simulink library "topr5_adapter"  (Simulink 8.2)
settings: Solver=ode1  StartTime=0.0  StopTime=Inf  FixedStep=0.001  RelTol=1e-3
PostLoadFcn:
  | , if any(exist('dsrtsu_mdlpostloadfcn', 'file') == [2, 3, 6]), try dsrtsu_mdlpostloadfcn('Execute', bdroot); catch fprintf('Error in PostLoadFcn (dsrtsu_mdlpostloadfcn) for model "%s":\n %s\n', bdroot, lasterr); end, end,
libraries: ParsingLibrary x32, simulink x4, srx_platform x3, topr5_adapter x2
settings Model: DSRTSU_INTERNAL_RTI_VER=450  DSRTSU_INTERNAL_RTI_TYPE=rti1401  DSRTSU_INTERNAL_RTIFPGA=40  Creator=leidos  LastModifiedBy=rushk1

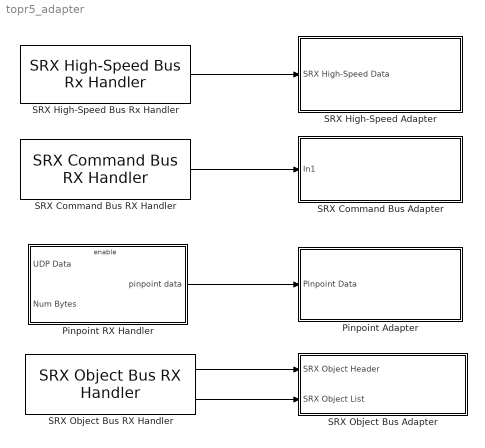
== system topr5_adapter ==
  Pinpoint Adapter : Subsystem
  Pinpoint RX Handler : Subsystem
  SRX Command Bus Adapter : Subsystem
  SRX Command Bus RX Handler : srx_platform/SRX Command Bus RX Handler  SystemSampleTime=-1
  SRX High-Speed Adapter : Subsystem
  SRX High-Speed Bus Rx Handler : srx_platform/SRX High-Speed Bus Rx Handler  SystemSampleTime=-1
  SRX Object Bus Adapter : Subsystem
  SRX Object Bus RX Handler : srx_platform/SRX Object Bus RX Handler
  wires:
  SRX Command Bus RX Handler/1 -> SRX Command Bus Adapter/1(In1)
  SRX High-Speed Bus Rx Handler/1 -> SRX High-Speed Adapter/1(SRX High-Speed Data)
  Pinpoint RX Handler/1(pinpoint data) -> Pinpoint Adapter/1(Pinpoint Data)
  SRX Object Bus RX Handler/1 -> SRX Object Bus Adapter/1(SRX Object Header)
  SRX Object Bus RX Handler/2 -> SRX Object Bus Adapter/2(SRX Object List)

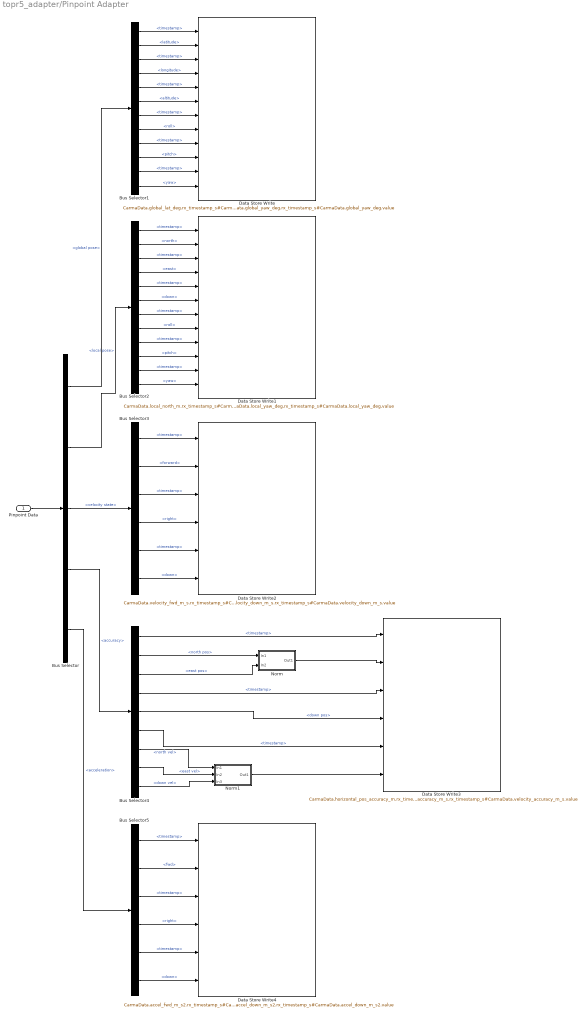
== system topr5_adapter/Pinpoint Adapter ==
  Pinpoint Data : Inport
  Bus Selector : BusSelector  OutputSignals=global pose,local pose,velocity state,accuracy,acceleration
  Bus Selector1 : BusSelector  OutputSignals=timestamp,latitude,timestamp,longitude,timestamp,altitude,timestamp,roll,timestamp,pitch,timestamp,yaw
  Bus Selector2 : BusSelector  OutputSignals=timestamp,north,timestamp,east,timestamp,down,timestamp,roll,timestamp,pitch,timestamp,yaw
  Bus Selector3 : BusSelector  OutputSignals=timestamp,forward,timestamp,right,timestamp,down
  Bus Selector4 : BusSelector  OutputSignals=timestamp,north pos,east pos,timestamp,down pos,timestamp,north vel,east vel,down vel
  Bus Selector5 : BusSelector  OutputSignals=timestamp,fwd,timestamp,right,timestamp,down
  Data Store Write : DataStoreWrite  DataStoreName=CarmaData  DataStoreElements=CarmaData.global_lat_deg.rx_timestamp_s#CarmaData.global_lat_deg.value#CarmaData.global_long_deg.rx_timestamp_s#CarmaData.global_long_deg.value#CarmaData.global_alt_m.rx_timestamp_s#CarmaData.global_alt_m.value#CarmaData.global_roll_deg.rx_timestamp_s#CarmaData.global_roll_deg.value#CarmaData.global_pitch_deg.rx_timestamp_s#CarmaData.global_pitch_deg.value#CarmaData.global_yaw_deg.rx_timestamp_s#CarmaData.global_yaw_deg.value
  Data Store Write1 : DataStoreWrite  DataStoreName=CarmaData  DataStoreElements=CarmaData.local_north_m.rx_timestamp_s#CarmaData.local_north_m.value#CarmaData.local_east_m.rx_timestamp_s#CarmaData.local_east_m.value#CarmaData.local_down_m.rx_timestamp_s#CarmaData.local_down_m.value#CarmaData.local_roll_deg.rx_timestamp_s#CarmaData.local_roll_deg.value#CarmaData.local_pitch_deg.rx_timestamp_s#CarmaData.local_pitch_deg.value#CarmaData.local_yaw_deg.rx_timestamp_s#CarmaData.local_yaw_deg.value
  Data Store Write2 : DataStoreWrite  DataStoreName=CarmaData  DataStoreElements=CarmaData.velocity_fwd_m_s.rx_timestamp_s#CarmaData.velocity_fwd_m_s.value#CarmaData.velocity_right_m_s.rx_timestamp_s#CarmaData.velocity_right_m_s.value#CarmaData.velocity_down_m_s.rx_timestamp_s#CarmaData.velocity_down_m_s.value
  Data Store Write3 : DataStoreWrite  DataStoreName=CarmaData  DataStoreElements=CarmaData.horizontal_pos_accuracy_m.rx_timestamp_s#CarmaData.horizontal_pos_accuracy_m.value#CarmaData.vertical_pos_accuracy_m.rx_timestamp_s#CarmaData.vertical_pos_accuracy_m.value#CarmaData.velocity_accuracy_m_s.rx_timestamp_s#CarmaData.velocity_accuracy_m_s.value
  Data Store Write4 : DataStoreWrite  DataStoreName=CarmaData  DataStoreElements=CarmaData.accel_fwd_m_s2.rx_timestamp_s#CarmaData.accel_fwd_m_s2.value#CarmaData.accel_right_m_s2.rx_timestamp_s#CarmaData.accel_right_m_s2.value#CarmaData.accel_down_m_s2.rx_timestamp_s#CarmaData.accel_down_m_s2.value
  Norm : Subsystem
  Norm1 : Subsystem
  wires:
  Bus Selector1/5 -> Data Store Write/5  "<timestamp>"
  Bus Selector1/3 -> Data Store Write/3  "<timestamp>"
  Bus Selector1/2 -> Data Store Write/2  "<latitude>"
  Bus Selector1/9 -> Data Store Write/9  "<timestamp>"
  Bus Selector1/6 -> Data Store Write/6  "<altitude>"
  Bus Selector1/7 -> Data Store Write/7  "<timestamp>"
  Bus Selector1/8 -> Data Store Write/8  "<roll>"
  Bus Selector1/11 -> Data Store Write/11  "<timestamp>"
  Bus Selector1/1 -> Data Store Write/1  "<timestamp>"
  Bus Selector1/4 -> Data Store Write/4  "<longitude>"
  Bus Selector1/10 -> Data Store Write/10  "<pitch>"
  Bus Selector1/12 -> Data Store Write/12  "<yaw>"
  Bus Selector5/3 -> Data Store Write4/3  "<timestamp>"
  Bus Selector5/2 -> Data Store Write4/2  "<fwd>"
  Bus Selector5/4 -> Data Store Write4/4  "<right>"
  Bus Selector5/6 -> Data Store Write4/6  "<down>"
  Bus Selector5/1 -> Data Store Write4/1  "<timestamp>"
  Bus Selector5/5 -> Data Store Write4/5  "<timestamp>"
  Bus Selector/5 -> Bus Selector5/1  "<acceleration>"
  Bus Selector4/6 -> Data Store Write3/5  "<timestamp>"
  Bus Selector4/5 -> Data Store Write3/4  "<down pos>"
  Bus Selector4/4 -> Data Store Write3/3  "<timestamp>"
  Bus Selector4/1 -> Data Store Write3/1  "<timestamp>"
  Bus Selector/4 -> Bus Selector4/1  "<accuracy>"
  Bus Selector3/6 -> Data Store Write2/6  "<down>"
  Bus Selector3/5 -> Data Store Write2/5  "<timestamp>"
  Bus Selector3/1 -> Data Store Write2/1  "<timestamp>"
  Bus Selector3/2 -> Data Store Write2/2  "<forward>"
  Bus Selector3/4 -> Data Store Write2/4  "<right>"
  Bus Selector3/3 -> Data Store Write2/3  "<timestamp>"
  Bus Selector/3 -> Bus Selector3/1  "<velocity state>"
  Bus Selector2/3 -> Data Store Write1/3  "<timestamp>"
  Bus Selector2/11 -> Data Store Write1/11  "<timestamp>"
  Bus Selector2/9 -> Data Store Write1/9  "<timestamp>"
  Bus Selector2/7 -> Data Store Write1/7  "<timestamp>"
  Bus Selector2/12 -> Data Store Write1/12  "<yaw>"
  Bus Selector2/5 -> Data Store Write1/5  "<timestamp>"
  Bus Selector2/6 -> Data Store Write1/6  "<down>"
  Bus Selector2/10 -> Data Store Write1/10  "<pitch>"
  Bus Selector2/8 -> Data Store Write1/8  "<roll>"
  Bus Selector2/4 -> Data Store Write1/4  "<east>"
  Bus Selector2/1 -> Data Store Write1/1  "<timestamp>"
  Bus Selector2/2 -> Data Store Write1/2  "<north>"
  Bus Selector/2 -> Bus Selector2/1  "<local pose>"
  Bus Selector/1 -> Bus Selector1/1  "<global pose>"
  Pinpoint Data/1 -> Bus Selector/1
  Norm1/1(Out1) -> Data Store Write3/6
  Bus Selector4/2 -> Norm/1(In1)  "<north pos>"
  Bus Selector4/3 -> Norm/2(In2)  "<east pos>"
  Norm/1(Out1) -> Data Store Write3/2
  Bus Selector4/7 -> Norm1/1(In1)  "<north vel>"
  Bus Selector4/8 -> Norm1/2(In2)  "<east vel>"
  Bus Selector4/9 -> Norm1/3(In3)  "<down vel>"

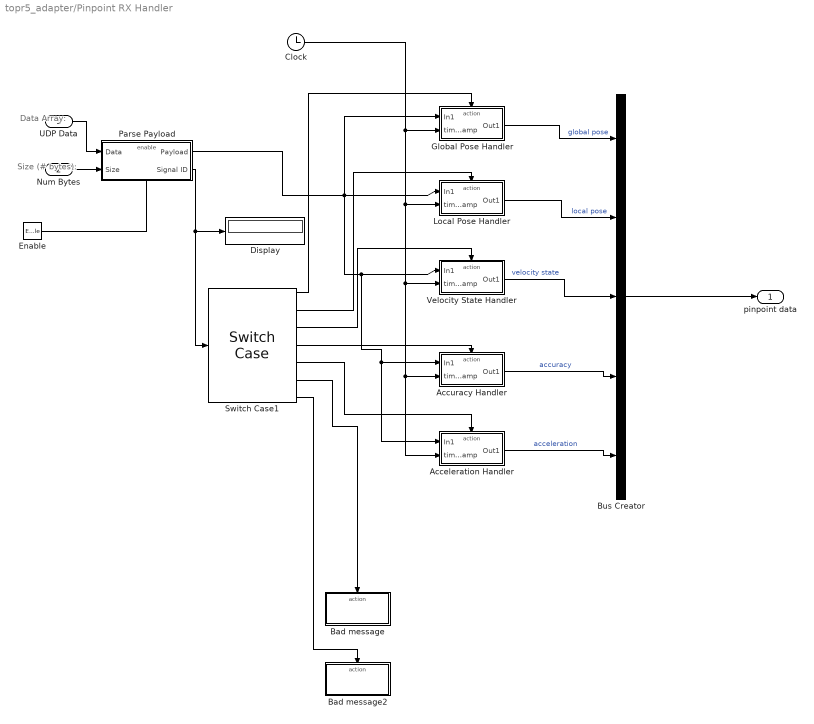
== system topr5_adapter/Pinpoint RX Handler ==
  note: Size (# bytes):
  note: Data Array:
  UDP Data : Inport  OutDataTypeStr=uint32  Interpolate=off
  Num Bytes : Inport  Port=2  OutDataTypeStr=int32
  Enable : EnablePort  PropagateVarSize=During execution  ShowOutputPort=on
  Acceleration Handler : Subsystem  TreatAsAtomicUnit=on
  Accuracy Handler : Subsystem  TreatAsAtomicUnit=on
  Bad message : Subsystem  TreatAsAtomicUnit=on
  Bad message2 : Subsystem  TreatAsAtomicUnit=on
  Bus Creator : BusCreator  Inputs=5
  Clock : Clock
  Display : Display
  Global Pose Handler : Subsystem  TreatAsAtomicUnit=on
  Local Pose Handler : Subsystem  TreatAsAtomicUnit=on
  Parse Payload : Subsystem  TreatAsAtomicUnit=on
  Switch Case1 : SwitchCase  CaseConditions={7, 9, 11, 6, 18, -1}
  Velocity State Handler : Subsystem  TreatAsAtomicUnit=on
  pinpoint data : Outport
  wires:
  Enable/1 -> Parse Payload/Enable
  Clock/1 -> Global Pose Handler/2(timestamp), Local Pose Handler/2(timestamp), Velocity State Handler/2(timestamp), Accuracy Handler/2(timestamp), Acceleration Handler/2(timestamp)
  Velocity State Handler/1(Out1) -> Bus Creator/3  "velocity state"
  Local Pose Handler/1(Out1) -> Bus Creator/2  "local pose"
  Global Pose Handler/1(Out1) -> Bus Creator/1  "global pose"
  Acceleration Handler/1(Out1) -> Bus Creator/5  "acceleration"
  Accuracy Handler/1(Out1) -> Bus Creator/4  "accuracy"
  Bus Creator/1 -> pinpoint data/1
  Switch Case1/6 -> Bad message/Action
  Switch Case1/4 -> Accuracy Handler/Action
  Switch Case1/5 -> Acceleration Handler/Action
  Switch Case1/1 -> Global Pose Handler/Action
  Switch Case1/7 -> Bad message2/Action
  Parse Payload/1(Payload) -> Accuracy Handler/1(In1), Acceleration Handler/1(In1), Velocity State Handler/1(In1), Global Pose Handler/1(In1), Local Pose Handler/1(In1)
  Switch Case1/2 -> Local Pose Handler/Action
  Switch Case1/3 -> Velocity State Handler/Action
  Parse Payload/2(Signal ID) -> Switch Case1/1, Display/1
  UDP Data/1 -> Parse Payload/1(Data)
  Num Bytes/1 -> Parse Payload/2(Size)

== system topr5_adapter/SRX Command Bus Adapter ==
  In1 : Inport
  Bus Selector : BusSelector  OutputSignals=UTC Time.UTC_Lower,UTC Time.UTC_Upper,UTC Time.time,Accel Module Feedback.AccelCmdInjectionFlag,Accel Module Feedback.time,Accel Module Feedback.AccelDriverOverride,Accel Module Feedback.time
  Data Store Write : DataStoreWrite  DataStoreName=CarmaData  DataStoreElements=CarmaData.global_utc_time_s.value#CarmaData.global_utc_time_s.rx_timestamp_s#CarmaData.path_ctrl_status.value#CarmaData.path_ctrl_status.rx_timestamp_s#CarmaData.throttle_ovr_flag.value#CarmaData.throttle_ovr_flag.rx_timestamp_s
  convert to double : Subsystem
  wires:
  In1/1 -> Bus Selector/1
  Bus Selector/3 -> Data Store Write/2  "<time>"
  Bus Selector/1 -> convert to double/1(In1)  "<UTC_Lower>"
  Bus Selector/2 -> convert to double/2(In2)  "<UTC_Upper>"
  convert to double/1(Out1) -> Data Store Write/1
  Bus Selector/5 -> Data Store Write/4  "<time>"
  Bus Selector/6 -> Data Store Write/5  "<AccelDriverOverride>"
  Bus Selector/7 -> Data Store Write/6  "<time>"
  Bus Selector/4 -> Data Store Write/3  "<AccelCmdInjectionFlag>"

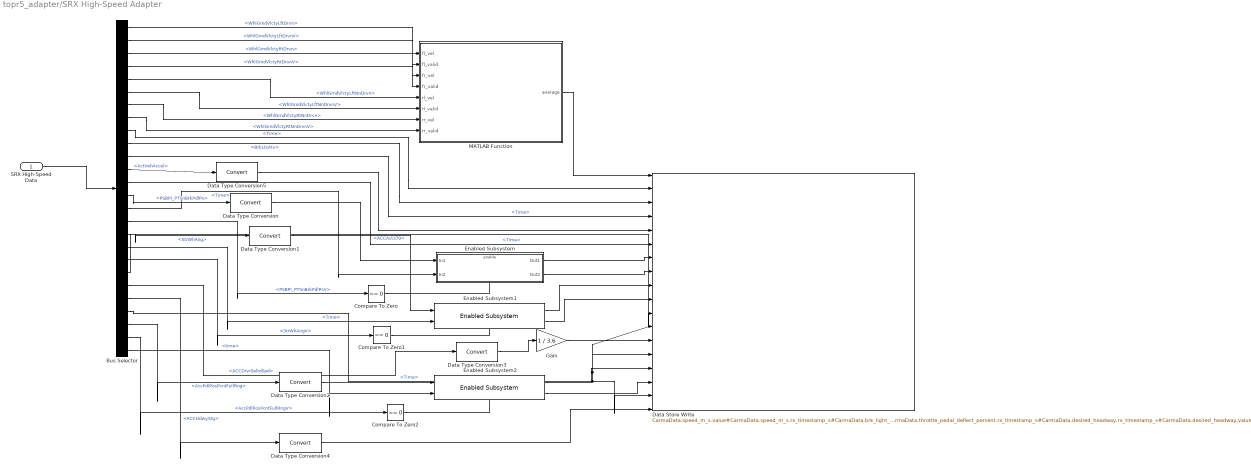
== system topr5_adapter/SRX High-Speed Adapter ==
  SRX High-Speed Data : Inport
  Bus Selector : BusSelector  OutputSignals="Front Wheel Velocity.WhlGrndVlctyLftDrvn,Front Wheel Velocity.WhlGrndVlctyLftDrvnV,Front Wheel Velocity.WhlGrndVlctyRtDrvn,Front Wheel Velocity.WhlGrndVlctyRtDrvnV,Rear Wheel  Velocity.WhlGrndVlctyLftNnDrvn,Rear Wheel  Velocity.WhlGrndVlctyLftNnDrvnV,Rear Wheel  Velocity.WhlGrndVlctyRtNnDrvn,Rear Wheel  Velocity.WhlGrndVlctyRtNnDrvnV,Front Wheel Velocity.Time,Exterior Lighting.BrkLtsAtv,Exterior Lighting.Time,Vehicle Accel.ActVehAccel,Vehicle Accel.Time,Brake Apply Status.PSBPI_PTSnBrkPdlPs,Brake Apply Status.Time,Brake Apply Status.PSBPI_PTSnBrkPdlPsV,Steering Wheel Angle.StrWhAng,Steering Wheel Angle.Time,Steering Wheel Angle.StrWhAngV,ACC Display Status .ACCAct370,ACC Display Status .ACCDrvrSeltdSpd,ACC Display Status .ACCHdwyStg,ACC Display Status .Time,Engine General Status.AccPdlPosPcntFullRng,Engine General Status.AccPdlPosPcntFullRngV,Engine General Status.time"
  Compare To Zero : simulink/Logic and Bit Operations/Compare To Zero  relop===  OutDataTypeStr=boolean
  Compare To Zero1 : simulink/Logic and Bit Operations/Compare To Zero  relop===  OutDataTypeStr=boolean
  Compare To Zero2 : simulink/Logic and Bit Operations/Compare To Zero  relop===  OutDataTypeStr=boolean
  Data Store Write : DataStoreWrite  DataStoreName=CarmaData  DataStoreElements=CarmaData.speed_m_s.value#CarmaData.speed_m_s.rx_timestamp_s#CarmaData.brk_light_flag.value#CarmaData.brk_light_flag.rx_timestamp_s#CarmaData.accel_m_s2.value#CarmaData.accel_m_s2.rx_timestamp_s#CarmaData.brk_pedal_deflect_percent.value#CarmaData.brk_pedal_deflect_percent.rx_timestamp_s#CarmaData.steering_wheel_angle_deg.value#CarmaData.steering_wheel_angle_deg.rx_timestamp_s#CarmaData.acc_status.value#CarmaData.acc_status.rx_timestamp_s#CarmaData.acc_set_speed_m_s.value#CarmaData.acc_set_speed_m_s.rx_timestamp_s#CarmaData.throttle_pedal_deflect_percent.value#CarmaData.throttle_pedal_deflect_percent.rx_timestamp_s#CarmaData.desired_headway.rx_timestamp_s#CarmaData.desired_headway.value
  Data Type Conversion{,1..5} (6 alike) : DataTypeConversion
  Enabled Subsystem : Subsystem  TreatAsAtomicUnit=on
  Enabled Subsystem1 : topr5_adapter/SRX High-Speed Adapter/Enabled Subsystem
  Enabled Subsystem2 : topr5_adapter/SRX High-Speed Adapter/Enabled Subsystem
  Gain : Gain  Gain=1 / 3.6
  MATLAB Function : MATLAB Function  TreatAsAtomicUnit=on
      settings: RTWSystemCode=Inline
  wires:
  SRX High-Speed Data/1 -> Bus Selector/1
  Bus Selector/1 -> MATLAB Function/1(fl_vel)  "<WhlGrndVlctyLftDrvn>"
  Bus Selector/2 -> MATLAB Function/2(fl_valid)  "<WhlGrndVlctyLftDrvnV>"
  Bus Selector/7 -> MATLAB Function/7(rr_vel)  "<WhlGrndVlctyRtNnDrvn>"
  Bus Selector/8 -> MATLAB Function/8(rr_valid)  "<WhlGrndVlctyRtNnDrvnV>"
  Bus Selector/3 -> MATLAB Function/3(fr_vel)  "<WhlGrndVlctyRtDrvn>"
  Bus Selector/4 -> MATLAB Function/4(fr_valid)  "<WhlGrndVlctyRtDrvnV>"
  Bus Selector/6 -> MATLAB Function/6(rl_valid)  "<WhlGrndVlctyLftNnDrvnV>"
  Bus Selector/5 -> MATLAB Function/5(rl_vel)  "<WhlGrndVlctyLftNnDrvn>"
  MATLAB Function/1(average) -> Data Store Write/1
  Bus Selector/9 -> Data Store Write/2  "<Time>"
  Bus Selector/10 -> Data Store Write/3  "<BrkLtsAtv>"
  Bus Selector/11 -> Data Store Write/4  "<Time>"
  Bus Selector/12 -> Data Type Conversion5/1  "<ActVehAccel>"
  Bus Selector/13 -> Data Store Write/6  "<Time>"
  Bus Selector/14 -> Data Type Conversion/1  "<PSBPI_PTSnBrkPdlPs>"
  Bus Selector/15 -> Enabled Subsystem/2(In2)  "<Time>"
  Bus Selector/16 -> Compare To Zero/1  "<PSBPI_PTSnBrkPdlPsV>"
  Bus Selector/17 -> Data Type Conversion1/1  "<StrWhAng>"
  Bus Selector/18 -> Enabled Subsystem1/2  "<Time>"
  Bus Selector/19 -> Compare To Zero1/1  "<StrWhAngV>"
  Bus Selector/20 -> Data Store Write/11  "<ACCAct370>"
  Bus Selector/23 -> Data Store Write/17, Data Store Write/14, Data Store Write/12  "<Time>"
  Data Type Conversion/1 -> Enabled Subsystem/1(In1)
  Data Type Conversion1/1 -> Enabled Subsystem1/1
  Compare To Zero/1 -> Enabled Subsystem/Enable
  Compare To Zero1/1 -> Enabled Subsystem1/Enable
  Enabled Subsystem/1(Out1) -> Data Store Write/7
  Enabled Subsystem/2(Out2) -> Data Store Write/8
  Enabled Subsystem1/1 -> Data Store Write/9
  Enabled Subsystem1/2 -> Data Store Write/10
  Bus Selector/24 -> Data Type Conversion2/1  "<AccPdlPosPcntFullRng>"
  Bus Selector/25 -> Compare To Zero2/1  "<AccPdlPosPcntFullRngV>"
  Bus Selector/26 -> Enabled Subsystem2/2  "<time>"
  Compare To Zero2/1 -> Enabled Subsystem2/Enable
  Enabled Subsystem2/1 -> Data Store Write/15
  Enabled Subsystem2/2 -> Data Store Write/16
  Data Type Conversion2/1 -> Enabled Subsystem2/1
  Bus Selector/21 -> Data Type Conversion3/1  "<ACCDrvrSeltdSpd>"
  Data Type Conversion3/1 -> Gain/1
  Bus Selector/22 -> Data Type Conversion4/1  "<ACCHdwyStg>"
  Data Type Conversion4/1 -> Data Store Write/18
  Data Type Conversion5/1 -> Data Store Write/5
  Gain/1 -> Data Store Write/13

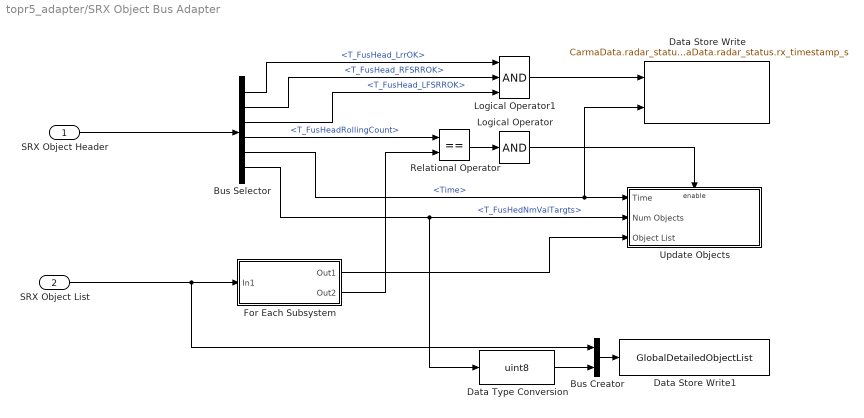
== system topr5_adapter/SRX Object Bus Adapter ==
  SRX Object Header : Inport
  SRX Object List : Inport  Port=2  OutDataTypeStr=Bus: FusObjectTrackA
  Bus Creator : BusCreator  Inputs=2  OutDataTypeStr=Bus: DetailedObjectList  NonVirtualBus=on
  Bus Selector : BusSelector  OutputSignals=T_FusHead_LrrOK,T_FusHead_RFSRROK,T_FusHead_LFSRROK,T_FusHeadRollingCount,Time,T_FusHedNmValTargts
  Data Store Write : DataStoreWrite  DataStoreName=CarmaData  DataStoreElements=CarmaData.radar_status.value#CarmaData.radar_status.rx_timestamp_s
  Data Store Write1 : DataStoreWrite  DataStoreName=GlobalDetailedObjectList
  Data Type Conversion : DataTypeConversion  OutDataTypeStr=uint8
  For Each Subsystem : Subsystem  TreatAsAtomicUnit=on
  Logical Operator : Logic  Inputs=1  AllPortsSameDT=off  OutDataTypeStr=boolean
  Logical Operator1 : Logic  Inputs=3  AllPortsSameDT=off  OutDataTypeStr=boolean
  Relational Operator : RelationalOperator  Operator===  OutDataTypeStr=boolean
  Update Objects : Subsystem
  wires:
  SRX Object Header/1 -> Bus Selector/1
  SRX Object List/1 -> Bus Creator/1, For Each Subsystem/1(In1)
  Bus Selector/4 -> Relational Operator/1  "<T_FusHeadRollingCount>"
  For Each Subsystem/2(Out2) -> Relational Operator/2
  Relational Operator/1 -> Logical Operator/1
  Bus Selector/5 -> Data Store Write/2, Update Objects/1(Time)  "<Time>"
  Bus Selector/6 -> Update Objects/2(Num Objects), Data Type Conversion/1  "<T_FusHedNmValTargts>"
  For Each Subsystem/1(Out1) -> Update Objects/3(Object List)
  Logical Operator/1 -> Update Objects/Enable
  Bus Selector/1 -> Logical Operator1/1  "<T_FusHead_LrrOK>"
  Bus Selector/3 -> Logical Operator1/3  "<T_FusHead_LFSRROK>"
  Bus Selector/2 -> Logical Operator1/2  "<T_FusHead_RFSRROK>"
  Logical Operator1/1 -> Data Store Write/1
  Bus Creator/1 -> Data Store Write1/1
  Data Type Conversion/1 -> Bus Creator/2

== system topr5_adapter/Pinpoint Adapter/Norm ==
  In1 : Inport
  In2 : Inport  Port=2
  Add : Sum
  Product : Product
  Product1 : Product
  Sqrt : Sqrt  SaturateOnIntegerOverflow=on
  Out1 : Outport
  wires:
  In2/1 -> Product1/1, Product1/2
  In1/1 -> Product/2, Product/1
  Add/1 -> Sqrt/1
  Product1/1 -> Add/2
  Sqrt/1 -> Out1/1
  Product/1 -> Add/1

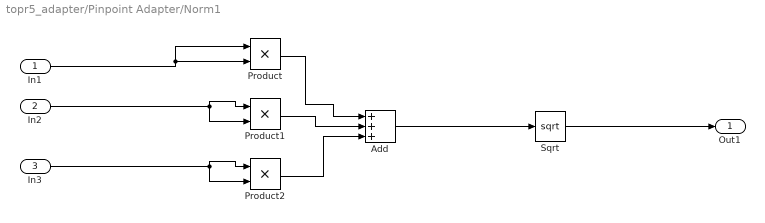
== system topr5_adapter/Pinpoint Adapter/Norm1 ==
  In1 : Inport
  In2 : Inport  Port=2
  In3 : Inport  Port=3
  Add : Sum  Inputs=+++
  Product : Product
  Product1 : Product
  Product2 : Product
  Sqrt : Sqrt  SaturateOnIntegerOverflow=on
  Out1 : Outport
  wires:
  In2/1 -> Product1/1, Product1/2
  In1/1 -> Product/2, Product/1
  Add/1 -> Sqrt/1
  Product1/1 -> Add/2
  Sqrt/1 -> Out1/1
  Product/1 -> Add/1
  In3/1 -> Product2/1, Product2/2
  Product2/1 -> Add/3

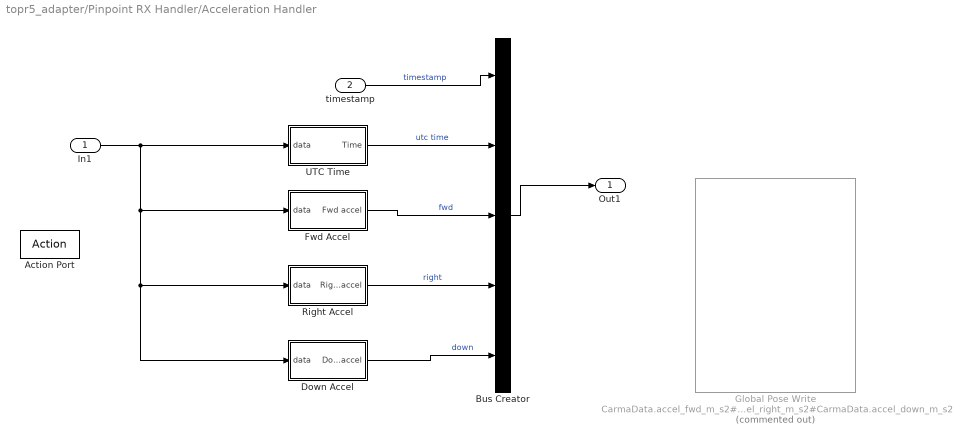
== system topr5_adapter/Pinpoint RX Handler/Acceleration Handler ==
  In1 : Inport
  timestamp : Inport  Port=2
  Action Port : ActionPort
  Bus Creator : BusCreator  Inputs=5
  Down Accel : Subsystem
  Fwd Accel : Subsystem
  Global Pose Write : DataStoreWrite  Commented=on  DataStoreName=CarmaData  DataStoreElements=CarmaData.accel_fwd_m_s2#CarmaData.accel_right_m_s2#CarmaData.accel_down_m_s2
  Right Accel : Subsystem
  UTC Time : Subsystem
  Out1 : Outport
  wires:
  Right Accel/1(Right accel) -> Bus Creator/4  "right"
  Fwd Accel/1(Fwd accel) -> Bus Creator/3  "fwd"
  Down Accel/1(Down accel) -> Bus Creator/5  "down"
  UTC Time/1(Time) -> Bus Creator/2  "utc time"
  timestamp/1 -> Bus Creator/1  "timestamp"
  Bus Creator/1 -> Out1/1
  In1/1 -> UTC Time/1(data), Fwd Accel/1(data), Right Accel/1(data), Down Accel/1(data)

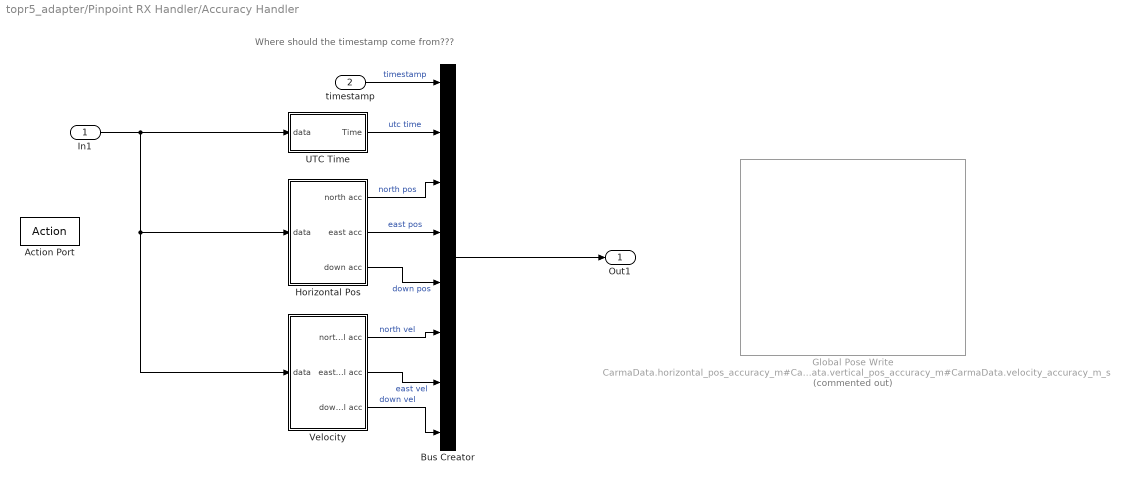
== system topr5_adapter/Pinpoint RX Handler/Accuracy Handler ==
  note: Where should the timestamp come from???
  In1 : Inport
  timestamp : Inport  Port=2
  Action Port : ActionPort
  Bus Creator : BusCreator  Inputs=8
  Global Pose Write : DataStoreWrite  Commented=on  DataStoreName=CarmaData  DataStoreElements=CarmaData.horizontal_pos_accuracy_m#CarmaData.vertical_pos_accuracy_m#CarmaData.velocity_accuracy_m_s
  Horizontal Pos : Subsystem
  UTC Time : Subsystem
  Velocity : Subsystem
  Out1 : Outport
  wires:
  Velocity/3(down vel acc) -> Bus Creator/8  "down vel"
  Horizontal Pos/3(down acc) -> Bus Creator/5  "down pos"
  Horizontal Pos/1(north acc) -> Bus Creator/3  "north pos"
  Velocity/2(east vel acc) -> Bus Creator/7  "east vel"
  Velocity/1(north vel acc) -> Bus Creator/6  "north vel"
  Horizontal Pos/2(east acc) -> Bus Creator/4  "east pos"
  UTC Time/1(Time) -> Bus Creator/2  "utc time"
  timestamp/1 -> Bus Creator/1  "timestamp"
  Bus Creator/1 -> Out1/1
  In1/1 -> UTC Time/1(data), Velocity/1(data), Horizontal Pos/1(data)

== system topr5_adapter/Pinpoint RX Handler/Bad message ==
  Action Port : ActionPort

== system topr5_adapter/Pinpoint RX Handler/Bad message2 ==
  Action Port : ActionPort

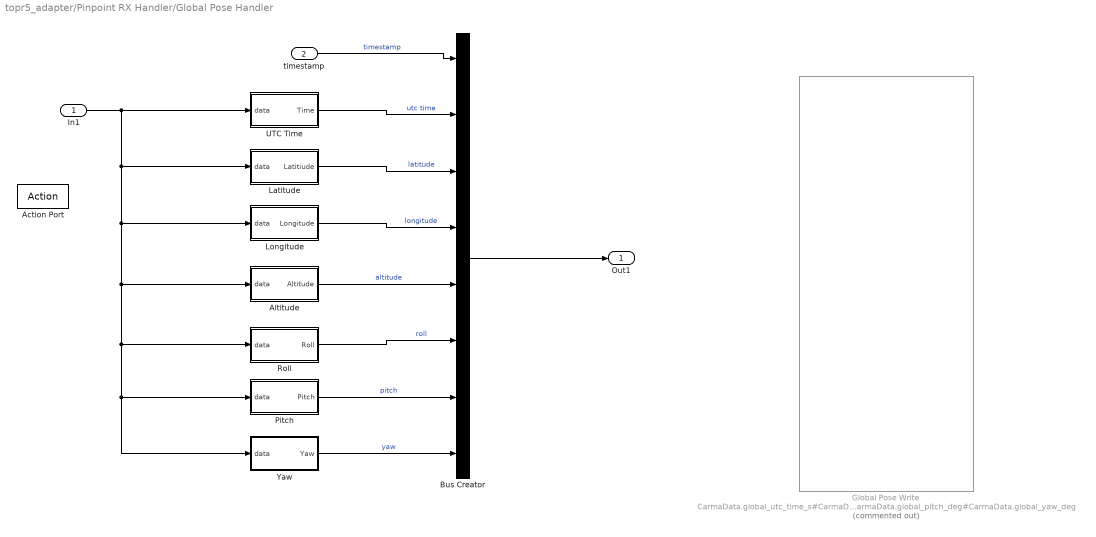
== system topr5_adapter/Pinpoint RX Handler/Global Pose Handler ==
  In1 : Inport
  timestamp : Inport  Port=2
  Action Port : ActionPort
  Altitude : Subsystem
  Bus Creator : BusCreator  Inputs=8
  Global Pose Write : DataStoreWrite  Commented=on  DataStoreName=CarmaData  DataStoreElements=CarmaData.global_utc_time_s#CarmaData.global_lat_deg#CarmaData.global_long_deg#CarmaData.global_alt_m#CarmaData.global_roll_deg#CarmaData.global_pitch_deg#CarmaData.global_yaw_deg
  Latitude : Subsystem
  Longitude : Subsystem
  Pitch : Subsystem
  Roll : Subsystem
  UTC Time : Subsystem
  Yaw : Subsystem
  Out1 : Outport
  wires:
  Bus Creator/1 -> Out1/1
  timestamp/1 -> Bus Creator/1  "timestamp"
  Latitude/1(Latitiude) -> Bus Creator/3  "latitude"
  UTC Time/1(Time) -> Bus Creator/2  "utc time"
  Roll/1(Roll) -> Bus Creator/6  "roll"
  Longitude/1(Longitude) -> Bus Creator/4  "longitude"
  Altitude/1(Altitude) -> Bus Creator/5  "altitude"
  Pitch/1(Pitch) -> Bus Creator/7  "pitch"
  Yaw/1(Yaw) -> Bus Creator/8  "yaw"
  In1/1 -> UTC Time/1(data), Latitude/1(data), Longitude/1(data), Altitude/1(data), Roll/1(data), Pitch/1(data), Yaw/1(data)

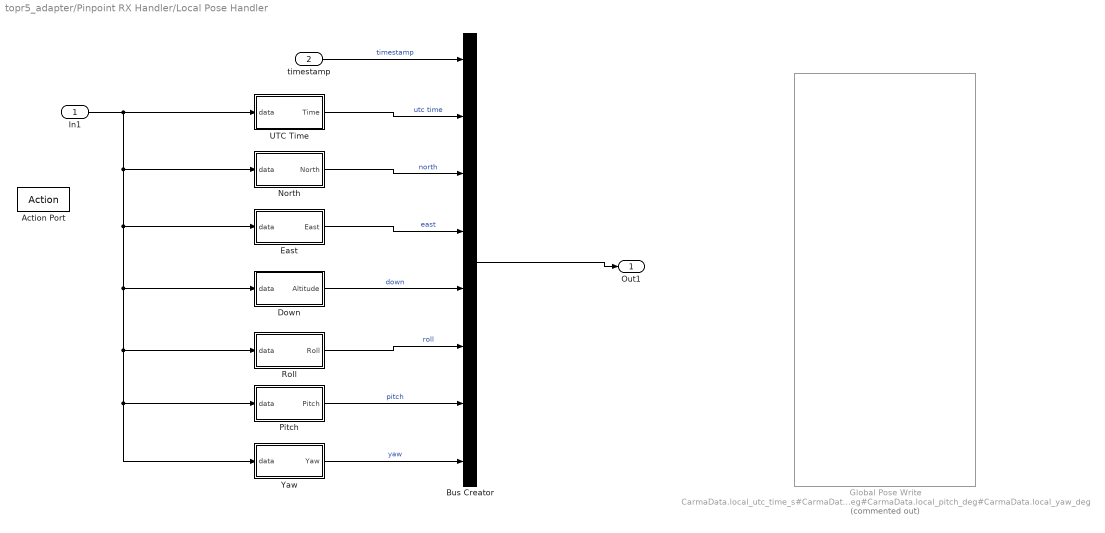
== system topr5_adapter/Pinpoint RX Handler/Local Pose Handler ==
  In1 : Inport
  timestamp : Inport  Port=2
  Action Port : ActionPort
  Bus Creator : BusCreator  Inputs=8
  Down : Subsystem
  East : Subsystem
  Global Pose Write : DataStoreWrite  Commented=on  DataStoreName=CarmaData  DataStoreElements=CarmaData.local_utc_time_s#CarmaData.local_north_m#CarmaData.local_east_m#CarmaData.local_down_m#CarmaData.local_roll_deg#CarmaData.local_pitch_deg#CarmaData.local_yaw_deg
  North : Subsystem
  Pitch : Subsystem
  Roll : Subsystem
  UTC Time : Subsystem
  Yaw : Subsystem
  Out1 : Outport
  wires:
  East/1(East) -> Bus Creator/4  "east"
  North/1(North) -> Bus Creator/3  "north"
  UTC Time/1(Time) -> Bus Creator/2  "utc time"
  Yaw/1(Yaw) -> Bus Creator/8  "yaw"
  Pitch/1(Pitch) -> Bus Creator/7  "pitch"
  Down/1(Altitude) -> Bus Creator/5  "down"
  Roll/1(Roll) -> Bus Creator/6  "roll"
  Bus Creator/1 -> Out1/1
  timestamp/1 -> Bus Creator/1  "timestamp"
  In1/1 -> UTC Time/1(data), North/1(data), East/1(data), Down/1(data), Roll/1(data), Pitch/1(data), Yaw/1(data)

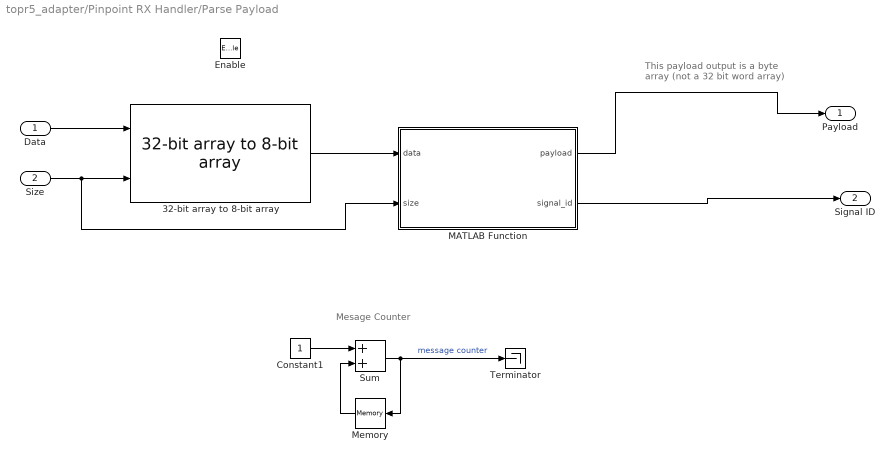
== system topr5_adapter/Pinpoint RX Handler/Parse Payload ==
  note: This payload output is a byte array
      | (not a 32 bit word array)
  note: Mesage Counter
  Data : Inport  OutDataTypeStr=uint32
  Size : Inport  Port=2  OutDataTypeStr=int32
  Enable : EnablePort  PropagateVarSize=During execution
  32-bit array to 8-bit array : ParsingLibrary/32-bit array to 8-bit array
  Constant1 : Constant
  MATLAB Function : MATLAB Function  TreatAsAtomicUnit=on
      settings: RTWSystemCode=Inline
  Memory : Memory  InheritSampleTime=on
  Sum : Sum  SaturateOnIntegerOverflow=on  InputSameDT=on  OutDataTypeStr=Inherit: Same as first input
  Terminator : Terminator
  Payload : Outport  OutDataTypeStr=uint8
  Signal ID : Outport  Port=2  OutDataTypeStr=uint8
  wires:
  Constant1/1 -> Sum/1
  Memory/1 -> Sum/2
  Sum/1 -> Memory/1, Terminator/1  "message counter"
  MATLAB Function/1(payload) -> Payload/1
  32-bit array to 8-bit array/1 -> MATLAB Function/1(data)
  Size/1 -> 32-bit array to 8-bit array/2, MATLAB Function/2(size)
  Data/1 -> 32-bit array to 8-bit array/1
  MATLAB Function/2(signal_id) -> Signal ID/1

== system topr5_adapter/Pinpoint RX Handler/Velocity State Handler ==
  In1 : Inport
  timestamp : Inport  Port=2
  Action Port : ActionPort
  Bus Creator : BusCreator  Inputs=5
  Down : Subsystem
  Fwd : Subsystem
  Right : Subsystem
  UTC Time : Subsystem
  Out1 : Outport
  wires:
  In1/1 -> UTC Time/1(data), Right/1(data), Down/1(data), Fwd/1(data)
  Right/1(right) -> Bus Creator/4  "right"
  Fwd/1(fwd) -> Bus Creator/3  "forward"
  UTC Time/1(Time) -> Bus Creator/2  "utc time"
  Down/1(down) -> Bus Creator/5  "down"
  Bus Creator/1 -> Out1/1
  timestamp/1 -> Bus Creator/1  "timestamp"

== system topr5_adapter/SRX Command Bus Adapter/convert to double ==
  In1 : Inport
  In2 : Inport  Port=2
  32-bit array to 8-bit array : ParsingLibrary/32-bit array to 8-bit array
  Constant : Constant  Value=8  OutDataTypeStr=uint32
  Mux : Mux  Inputs=2
  Parse 64 bit int : ParsingLibrary/Parse 64 bit int  Value=[0:7]  factor=1 / 1000000  OutDataTypeStr=double
  Out1 : Outport
  wires:
  32-bit array to 8-bit array/1 -> Parse 64 bit int/1
  Parse 64 bit int/1 -> Out1/1
  Constant/1 -> 32-bit array to 8-bit array/2
  In1/1 -> Mux/1
  In2/1 -> Mux/2
  Mux/1 -> 32-bit array to 8-bit array/1

== system topr5_adapter/SRX High-Speed Adapter/Enabled Subsystem ==
  In1 : Inport
  In2 : Inport  Port=2
  Enable : EnablePort
  Out1 : Outport
  Out2 : Outport  Port=2
  wires:
  In1/1 -> Out1/1
  In2/1 -> Out2/1

== system topr5_adapter/SRX Object Bus Adapter/For Each Subsystem ==
  In1 : Inport  Partition=on  PartitionDimension=1  PartitionWidth=1
  Bus Creator : BusCreator  Inputs=2  OutDataTypeStr=Bus: FusObjectData  NonVirtualBus=on
  Bus Selector : BusSelector  OutputSignals=FwdFusTrkALongPos,FwdFusTrkARelLongVel,FwdFusTrkARollingCnt
  For Each : ForEach  DisableCoverage=on  IndexMode=One-based
  Out1 : Outport  ConcatenationDimension=1
  Out2 : Outport  Port=2  ConcatenationDimension=1
  wires:
  In1/1 -> Bus Selector/1
  Bus Selector/1 -> Bus Creator/1  "<FwdFusTrkALongPos>"
  Bus Selector/2 -> Bus Creator/2  "<FwdFusTrkARelLongVel>"
  Bus Creator/1 -> Out1/1
  Bus Selector/3 -> Out2/1  "<FwdFusTrkARollingCnt>"

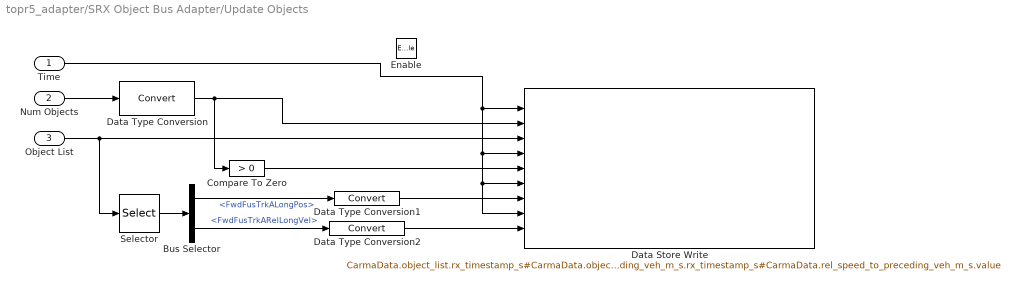
== system topr5_adapter/SRX Object Bus Adapter/Update Objects ==
  Time : Inport
  Num Objects : Inport  Port=2
  Object List : Inport  Port=3
  Enable : EnablePort
  Bus Selector : BusSelector  OutputSignals=FwdFusTrkALongPos,FwdFusTrkARelLongVel
  Compare To Zero : simulink/Logic and Bit Operations/Compare To Zero  relop=>  OutDataTypeStr=boolean
  Data Store Write : DataStoreWrite  DataStoreName=CarmaData  DataStoreElements=CarmaData.object_list.rx_timestamp_s#CarmaData.object_list.value.num_objects#CarmaData.object_list.value.object_list(:)#CarmaData.preceding_veh_flag.rx_timestamp_s#CarmaData.preceding_veh_flag.value#CarmaData.dist_to_preceding_veh_m.rx_timestamp_s#CarmaData.dist_to_preceding_veh_m.value#CarmaData.rel_speed_to_preceding_veh_m_s.rx_timestamp_s#CarmaData.rel_speed_to_preceding_veh_m_s.value
  Data Type Conversion : DataTypeConversion
  Data Type Conversion1 : DataTypeConversion
  Data Type Conversion2 : DataTypeConversion
  Selector : Selector  InputPortWidth=4  IndexOptions=Index vector (dialog)  Indices=[1]  OutputSizes=1
  wires:
  Time/1 -> Data Store Write/8, Data Store Write/6, Data Store Write/4, Data Store Write/1
  Object List/1 -> Selector/1, Data Store Write/3
  Num Objects/1 -> Data Type Conversion/1
  Data Type Conversion/1 -> Compare To Zero/1, Data Store Write/2
  Compare To Zero/1 -> Data Store Write/5
  Selector/1 -> Bus Selector/1
  Bus Selector/1 -> Data Type Conversion1/1  "<FwdFusTrkALongPos>"
  Bus Selector/2 -> Data Type Conversion2/1  "<FwdFusTrkARelLongVel>"
  Data Type Conversion1/1 -> Data Store Write/7
  Data Type Conversion2/1 -> Data Store Write/9

== system topr5_adapter/Pinpoint RX Handler/Acceleration Handler/Down Accel ==
  data : Inport
  Parse 16 bit int : ParsingLibrary/Parse 16 bit int  Value=[12:13]  InDataTypeStr=int16  factor=1 / 1000  OutDataTypeStr=single
  Down accel : Outport
  wires:
  data/1 -> Parse 16 bit int/1
  Parse 16 bit int/1 -> Down accel/1

== system topr5_adapter/Pinpoint RX Handler/Acceleration Handler/Fwd Accel ==
  data : Inport
  Parse 16 bit int : ParsingLibrary/Parse 16 bit int  Value=[8:9]  InDataTypeStr=int16  factor=1 / 1000  OutDataTypeStr=single
  Fwd accel : Outport
  wires:
  data/1 -> Parse 16 bit int/1
  Parse 16 bit int/1 -> Fwd accel/1

== system topr5_adapter/Pinpoint RX Handler/Acceleration Handler/Right Accel ==
  data : Inport
  Parse 16 bit int : ParsingLibrary/Parse 16 bit int  Value=[10:11]  InDataTypeStr=int16  factor=1 / 1000  OutDataTypeStr=single
  Right accel : Outport
  wires:
  data/1 -> Parse 16 bit int/1
  Parse 16 bit int/1 -> Right accel/1

== system topr5_adapter/Pinpoint RX Handler/Acceleration Handler/UTC Time ==
  data : Inport
  Parse 64 bit : ParsingLibrary/Parse 64 bit int  Value=[0:7]  factor=1 / 1000000  OutDataTypeStr=double
  Time : Outport
  wires:
  Parse 64 bit/1 -> Time/1
  data/1 -> Parse 64 bit/1

== system topr5_adapter/Pinpoint RX Handler/Accuracy Handler/Horizontal Pos ==
  note: NORTH:
  note: EAST:
  note: DOWN:
  data : Inport
  Parse 32 bit single : ParsingLibrary/Parse 32 bit single  Value=[8:11]  Flip=true  factor=1  OutDataTypeStr=single
  Parse 32 bit single1 : ParsingLibrary/Parse 32 bit single  Value=[12:15]  Flip=true  factor=1  OutDataTypeStr=single
  Parse 32 bit single2 : ParsingLibrary/Parse 32 bit single  Value=[16:19]  Flip=true  factor=1  OutDataTypeStr=single
  north acc : Outport
  east acc : Outport  Port=2
  down acc : Outport  Port=3
  wires:
  Parse 32 bit single2/1 -> down acc/1
  Parse 32 bit single1/1 -> east acc/1
  Parse 32 bit single/1 -> north acc/1
  data/1 -> Parse 32 bit single/1, Parse 32 bit single1/1, Parse 32 bit single2/1

== system topr5_adapter/Pinpoint RX Handler/Accuracy Handler/UTC Time ==
  data : Inport
  Parse 64 bit : ParsingLibrary/Parse 64 bit int  Value=[0:7]  factor=1 / 1000000  OutDataTypeStr=double
  Time : Outport
  wires:
  Parse 64 bit/1 -> Time/1
  data/1 -> Parse 64 bit/1

== system topr5_adapter/Pinpoint RX Handler/Accuracy Handler/Velocity ==
  note: North:
  note: East
  note: Down
  note: Outputs the max between north velocity, east velocity,
      | and down velocity accuracies
  data : Inport
  Parse 32 bit single : ParsingLibrary/Parse 32 bit single  Value=[20:23]  Flip=true  factor=1  OutDataTypeStr=single
  Parse 32 bit single1 : ParsingLibrary/Parse 32 bit single  Value=[24:27]  Flip=true  factor=1  OutDataTypeStr=single
  Parse 32 bit single2 : ParsingLibrary/Parse 32 bit single  Value=[28:31]  Flip=true  factor=1  OutDataTypeStr=single
  north vel acc : Outport
  east vel acc : Outport  Port=2
  down vel acc : Outport  Port=3
  wires:
  Parse 32 bit single2/1 -> down vel acc/1
  Parse 32 bit single1/1 -> east vel acc/1
  Parse 32 bit single/1 -> north vel acc/1
  data/1 -> Parse 32 bit single/1, Parse 32 bit single1/1, Parse 32 bit single2/1

== system topr5_adapter/Pinpoint RX Handler/Global Pose Handler/Altitude ==
  data : Inport
  Parse 32 bit : ParsingLibrary/Parse 32 bit int  Value2=[16:19]  OutDataTypeStr=double  InDataTypeStr=int32  Value=1/1000
  Altitude : Outport
  wires:
  Parse 32 bit/1 -> Altitude/1
  data/1 -> Parse 32 bit/1

== system topr5_adapter/Pinpoint RX Handler/Global Pose Handler/Latitude ==
  data : Inport
  Parse 32 bit : ParsingLibrary/Parse 32 bit int  Value2=[8:11]  OutDataTypeStr=double  InDataTypeStr=int32  Value=180.0 / 2^31
  Latitiude : Outport
  wires:
  data/1 -> Parse 32 bit/1
  Parse 32 bit/1 -> Latitiude/1

== system topr5_adapter/Pinpoint RX Handler/Global Pose Handler/Longitude ==
  data : Inport
  Parse 32 bit : ParsingLibrary/Parse 32 bit int  Value2=[12:15]  OutDataTypeStr=double  InDataTypeStr=int32  Value=180.0 / 2^31
  Longitude : Outport
  wires:
  data/1 -> Parse 32 bit/1
  Parse 32 bit/1 -> Longitude/1

== system topr5_adapter/Pinpoint RX Handler/Global Pose Handler/Pitch ==
  data : Inport
  Parse 16 bit : ParsingLibrary/Parse 16 bit int  Value=[22:23]  InDataTypeStr=int16  factor=180 / 2^15  OutDataTypeStr=single
  Pitch : Outport
  wires:
  Parse 16 bit/1 -> Pitch/1
  data/1 -> Parse 16 bit/1

== system topr5_adapter/Pinpoint RX Handler/Global Pose Handler/Roll ==
  data : Inport
  Parse 16 bit : ParsingLibrary/Parse 16 bit int  Value=[20:21]  InDataTypeStr=int16  factor=180 / 2^15  OutDataTypeStr=single
  Roll : Outport
  wires:
  Parse 16 bit/1 -> Roll/1
  data/1 -> Parse 16 bit/1

== system topr5_adapter/Pinpoint RX Handler/Global Pose Handler/UTC Time ==
  data : Inport
  Parse 64 bit : ParsingLibrary/Parse 64 bit int  Value=[0:7]  factor=1 / 1000000  OutDataTypeStr=double
  Time : Outport
  wires:
  Parse 64 bit/1 -> Time/1
  data/1 -> Parse 64 bit/1

== system topr5_adapter/Pinpoint RX Handler/Global Pose Handler/Yaw ==
  data : Inport
  Parse 16 bit : ParsingLibrary/Parse 16 bit int  Value=[24:25]  InDataTypeStr=int16  factor=180 / 2^15  OutDataTypeStr=single
  Yaw : Outport
  wires:
  Parse 16 bit/1 -> Yaw/1
  data/1 -> Parse 16 bit/1

== system topr5_adapter/Pinpoint RX Handler/Local Pose Handler/Down ==
  data : Inport
  Parse 32 bit : ParsingLibrary/Parse 32 bit int  Value2=[16:19]  OutDataTypeStr=double  InDataTypeStr=int32  Value=1/1000
  Altitude : Outport
  wires:
  Parse 32 bit/1 -> Altitude/1
  data/1 -> Parse 32 bit/1

== system topr5_adapter/Pinpoint RX Handler/Local Pose Handler/East ==
  data : Inport
  Parse 32 bit : ParsingLibrary/Parse 32 bit int  Value2=[12:15]  OutDataTypeStr=double  InDataTypeStr=int32  Value=1 / 1000
  East : Outport
  wires:
  data/1 -> Parse 32 bit/1
  Parse 32 bit/1 -> East/1

== system topr5_adapter/Pinpoint RX Handler/Local Pose Handler/North ==
  data : Inport
  Parse 32 bit : ParsingLibrary/Parse 32 bit int  Value2=[8:11]  OutDataTypeStr=double  InDataTypeStr=int32  Value=1 / 1000
  North : Outport
  wires:
  data/1 -> Parse 32 bit/1
  Parse 32 bit/1 -> North/1

== system topr5_adapter/Pinpoint RX Handler/Local Pose Handler/Pitch ==
  data : Inport
  Parse 16 bit : ParsingLibrary/Parse 16 bit int  Value=[22:23]  InDataTypeStr=int16  factor=180 / 2^15  OutDataTypeStr=single
  Pitch : Outport
  wires:
  Parse 16 bit/1 -> Pitch/1
  data/1 -> Parse 16 bit/1

== system topr5_adapter/Pinpoint RX Handler/Local Pose Handler/Roll ==
  data : Inport
  Parse 16 bit : ParsingLibrary/Parse 16 bit int  Value=[20:21]  InDataTypeStr=int16  factor=180 / 2^15  OutDataTypeStr=single
  Roll : Outport
  wires:
  Parse 16 bit/1 -> Roll/1
  data/1 -> Parse 16 bit/1

== system topr5_adapter/Pinpoint RX Handler/Local Pose Handler/UTC Time ==
  data : Inport
  Parse 64 bit : ParsingLibrary/Parse 64 bit int  Value=[0:7]  factor=1 / 1000000  OutDataTypeStr=double
  Time : Outport
  wires:
  Parse 64 bit/1 -> Time/1
  data/1 -> Parse 64 bit/1

== system topr5_adapter/Pinpoint RX Handler/Local Pose Handler/Yaw ==
  data : Inport
  Parse 16 bit : ParsingLibrary/Parse 16 bit int  Value=[24:25]  InDataTypeStr=int16  factor=180 / 2^15  OutDataTypeStr=single
  Yaw : Outport
  wires:
  Parse 16 bit/1 -> Yaw/1
  data/1 -> Parse 16 bit/1

== system topr5_adapter/Pinpoint RX Handler/Velocity State Handler/Down ==
  data : Inport
  Parse 24 bit int : ParsingLibrary/Parse 24 bit int  Value2=[14:16]  OutDataTypeStr=single  InDataTypeStr=int32  Value=1 / 1000
  down : Outport
  wires:
  Parse 24 bit int/1 -> down/1
  data/1 -> Parse 24 bit int/1

== system topr5_adapter/Pinpoint RX Handler/Velocity State Handler/Fwd ==
  data : Inport
  Parse 24 bit int : ParsingLibrary/Parse 24 bit int  Value2=[8:10]  OutDataTypeStr=single  InDataTypeStr=int32  Value=1 / 1000
  fwd : Outport
  wires:
  data/1 -> Parse 24 bit int/1
  Parse 24 bit int/1 -> fwd/1

== system topr5_adapter/Pinpoint RX Handler/Velocity State Handler/Right ==
  data : Inport
  Parse 24 bit int : ParsingLibrary/Parse 24 bit int  Value2=[11:13]  OutDataTypeStr=single  InDataTypeStr=int32  Value=1 / 1000
  right : Outport
  wires:
  data/1 -> Parse 24 bit int/1
  Parse 24 bit int/1 -> right/1

== system topr5_adapter/Pinpoint RX Handler/Velocity State Handler/UTC Time ==
  data : Inport
  Parse 64 bit : ParsingLibrary/Parse 64 bit int  Value=[0:7]  factor=1 / 1000000  OutDataTypeStr=double
  Time : Outport
  wires:
  Parse 64 bit/1 -> Time/1
  data/1 -> Parse 64 bit/1

== matlab function Pinpoint RX Handler/Parse Payload/MATLAB Function ==
  data: payload output uint8 size=[1 1472]; signal_id output double; data input double; size input double
% IN:
% data - array of bytes containing UDP packet data. May contain padding at
%        the end
% size - signed 32 bit integer representing the number of bytes in the actual UDP
%        message
%
% OUT:
% payload - array of 8-bit unsigned integers contiaining the payload of the
%           message
% type    - 8-bit unsigned integer representing the message ID of the
%           payload data (each pinpoint message has a unique id)

function [payload, signal_id]= parseScheduledReturn(data, size)
%#codegen

% payload = zeros(1,60, 'uint8'); % 60 bytes should be larger than any pinpt message
signal_id = uint8(-1);

%Constants
HEADER_SIZE = 2;
MSGTYPE_SIGNAL_EMITTED = 3;
MSGTYPE_SCHEDULE_RETURN = 4;


% Make sure there's enough data for the header
if size < HEADER_SIZE
    payload = uint8(0);
    fprintf('Not enough data for header\r\n');
    return
end
controlbyte = uint8(data(1)); % pull out the first byte
signal_id = uint8(data(2)); % pull out second byte
fprintf('Signal ID: %i\r\n', int32(signal_id));

% check for (and ignore) a protocol message
if bitand(controlbyte, 128) > 0 %bit 7
    signal_id = uint8(-1);
    payload = uint8(0);
    fprintf('Protocol Message\r\n');
    return
end

% Ignore anything that's not a schedule return message
if bitand(bitshift(controlbyte, -3), 15) ~= MSGTYPE_SCHEDULE_RETURN %bits 6:3
    signal_id = uint8(-1);
    payload = uint8(0);
    fprintf('Non-signal message\r\n');
    return
end

size_enum = bitand(controlbyte, 3); % 0: no data, 1: single byte size, 2: 2 two byte size, 3: 4 byte size

% payload_size = uint32(0);
payload_start = 3;

if size_enum == 1
    payload_size = uint32(data(3)); %third byte
    payload_start = payload_start + 1;
    HEADER_SIZE = HEADER_SIZE + 1;
elseif size_enum == 2
    payload_size = uint32(bitor(bitshift(uint16(data(4)), 8), uint16(data(3)))); %third and fourth bytes
    payload_start = payload_start + 2;
    HEADER_SIZE = HEADER_SIZE + 2;
elseif size_enum == 3
    payload_size = bitor(bitshift(uint32(data(4)), 8), uint32(data(3))); %third and fourth bytes
    payload_size = bitor(uint32(payload_size), bitor(bitshift(uint32(data(6)), 24), bitshift(uint32(data(5)), 16))); %first & second bytes of second integer
    payload_start = payload_start + 4;
    HEADER_SIZE = HEADER_SIZE + 4;
else
    signal_id = uint8(-1);
    payload = uint8(0);
    fprintf('Bad size enum (%i)\r\n', int32(size_enum));
    return
end

fprintf('Payload size: %i\r\n', int32(payload_size));
% make sure there's enough data to fill in the payload
if payload_size > (size - HEADER_SIZE)
    signal_id = uint8(-1);
    payload = uint8(0);
    fprintf('Not enough payload\r\n');
    return
end

payload = data(payload_start:payload_start+payload_size-1);
    
end

== matlab function SRX High-Speed Adapter/MATLAB Function ==
  data: fl_vel input double; average output single; fl_valid input double; fr_vel input double; fr_valid input double; rl_vel input double; rl_valid input double; rr_vel input double; rr_valid input double
function average = avg_wheelspeeds(fl_vel, fl_valid, fr_vel, fr_valid,... 
    rl_vel, rl_valid, rr_vel, rr_valid)
%#codegen
speed_sum = 0;
value_total = 0;

% Valid flags seem to always be zero, (which is why they're commented out)
if (~fl_valid)
    value_total = value_total + 1;
    speed_sum = speed_sum + fl_vel;
end
if (~fr_valid)
    value_total = value_total + 1;
    speed_sum = speed_sum + fr_vel;
end
if (~rl_valid)
    value_total = value_total + 1;
    speed_sum = speed_sum + rl_vel;
end
if (~rr_valid)
    value_total = value_total + 1;
    speed_sum = speed_sum + rr_vel;
end
if (speed_sum == 0)
    average = single(0);
else
    average = single((speed_sum/value_total) / 3.6);
end
